simulink model "lab_2_sim"  (R2021a)
settings: Solver=VariableStepAuto  StartTime=0.0  StopTime=10.0  RelTol=1e-3
values from neighbouring files (symbols this model uses):
  B_sm = 20e3    (= 20000)    [lab_2_sm.m]
  K_sm = 1    [lab_2_sm.m]
settings Model: Creator=Ahmed  LastModifiedBy=Ahmed

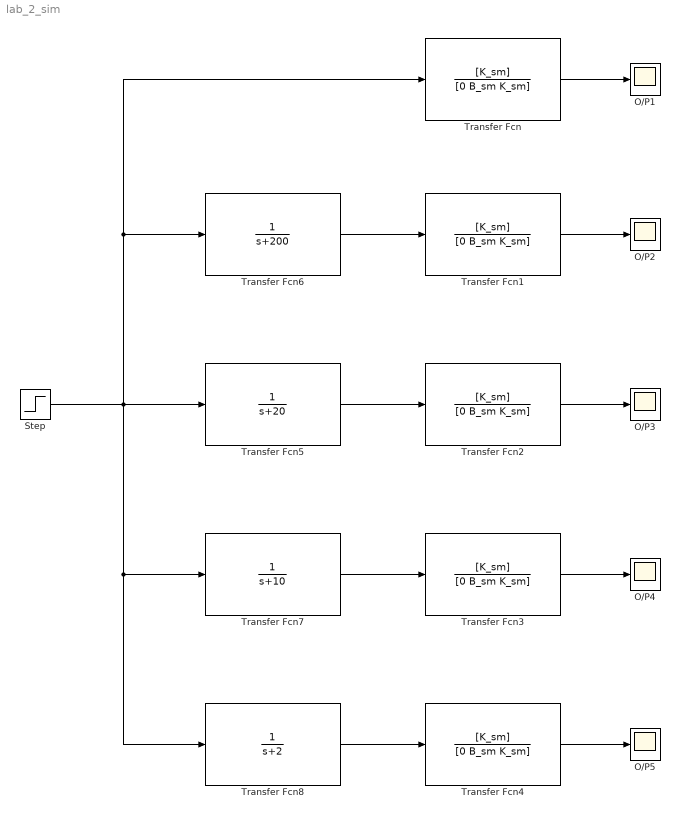
== system lab_2_sim ==
  O/P{1..5} (5 alike) : Scope
  Step : Step  Time=0  SampleTime=0
  Transfer Fcn{,1..4} (5 alike) : TransferFcn  Numerator=[K_sm]  Denominator=[0 B_sm K_sm]
  Transfer Fcn5 : TransferFcn  Numerator=[0 1]  Denominator=[1 20]
  Transfer Fcn6 : TransferFcn  Numerator=[0 1]  Denominator=[1 200]
  Transfer Fcn7 : TransferFcn  Numerator=[0 1]  Denominator=[1 10]
  Transfer Fcn8 : TransferFcn  Numerator=[0 1]  Denominator=[1 2]
  wires:
  Transfer Fcn/1 -> O/P1/1
  Transfer Fcn1/1 -> O/P2/1
  Transfer Fcn2/1 -> O/P3/1
  Transfer Fcn3/1 -> O/P4/1
  Transfer Fcn4/1 -> O/P5/1
  Transfer Fcn8/1 -> Transfer Fcn4/1
  Transfer Fcn6/1 -> Transfer Fcn1/1
  Transfer Fcn5/1 -> Transfer Fcn2/1
  Transfer Fcn7/1 -> Transfer Fcn3/1
  Step/1 -> Transfer Fcn8/1, Transfer Fcn7/1, Transfer Fcn6/1, Transfer Fcn/1, Transfer Fcn5/1
